simulink model "CalebsLaunchControl"  (R2019b)
settings: Solver=ode1  StartTime=0.0  StopTime=inf  FixedStep=0.0002  RelTol=1e-3
PreLoadFcn:
  | vehicle = 'Car'; if ~length(which('cmself')), cmenv; end
  | CalebsLaunchControl_bus
InitFcn:
  | vehicle = 'Car'; if ~length(which('cmself')), cmenv; end
  | CalebsLaunchControl_bus
model workspace (MAT data in the model file):
  LC_REVRANGE = [0 400 800 1200 1600 2000 3000 4000 6000 22000]
  MotorData = [0 4 8 13 17 21 0 4 8 13 17 21 ... (84 elements, 6x14)]
  POWER_AT_FULL_GAS = [21 21 21 21 21 21 21 21 21 20 20 19 ... (14 elements, 1x14)]
  RPM_RANGE = [0 2000 4000 6000 8000 10000 12000 14000 15000 16000 17000 18000 ... (14 elements, 1x14)]
  TC_MODE_ONE = [18 20 23 25 25 25 25 25 25 25]
  TC_MODE_ONE_FRONT = [9 10 12 15 25 25 25 25 25 25 25 25 ... (14 elements, 1x14)]
  ThrottleOpening = [0 0.2 0.4 0.6 0.8 1]
libraries: CarMaker4SL x8
(part 2 of 2)

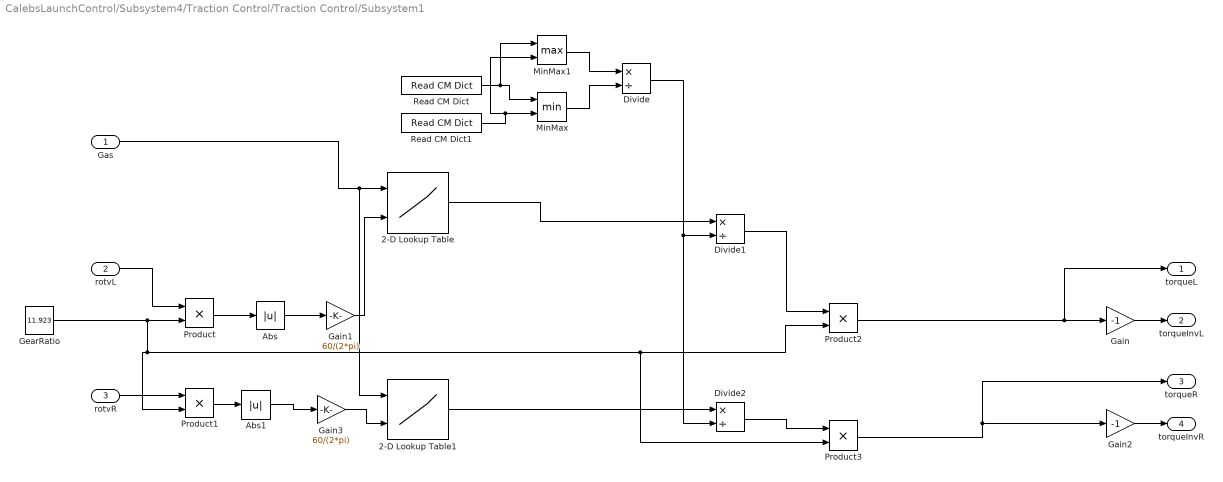
== system CalebsLaunchControl/Subsystem4/Traction Control/Traction Control/Subsystem1 ==
  Gas : Inport
  rotvL : Inport  Port=2
  rotvR : Inport  Port=3
  2-D Lookup Table : Lookup_n-D  BreakpointsForDimension1=ThrottleOpening  BreakpointsForDimension2=RPM_RANGE  Table=MotorData  InternalRulePriority=Speed  RndMeth=Simplest  InputSameDT=on
  2-D Lookup Table1 : Lookup_n-D  BreakpointsForDimension1=ThrottleOpening  BreakpointsForDimension2=RPM_RANGE  Table=MotorData  InternalRulePriority=Speed  RndMeth=Simplest  InputSameDT=on
  Abs : Abs
  Abs1 : Abs
  Divide : Product  Inputs=*/
  Divide1 : Product  Inputs=*/
  Divide2 : Product  Inputs=*/
  Gain : Gain  Gain=-1
  Gain1 : Gain  Gain=60/(2*pi)
  Gain2 : Gain  Gain=-1
  Gain3 : Gain  Gain=60/(2*pi)
  GearRatio : Constant  Value=11.923
  MinMax : MinMax  Inputs=2
  MinMax1 : MinMax  Function=max  Inputs=2
  Product{,1..3} (4 alike) : Product
  Read CM Dict : CarMaker4SL/Read CM Dict  xname=Car.LongSlipRL  xsync=off
  Read CM Dict1 : CarMaker4SL/Read CM Dict  xname=Car.LongSlipRR  xsync=off
  torqueL : Outport
  torqueInvL : Outport  Port=2
  torqueR : Outport  Port=3
  torqueInvR : Outport  Port=4
  wires:
  Gain/1 -> torqueInvL/1
  Product/1 -> Abs/1
  Gas/1 -> 2-D Lookup Table1/1, 2-D Lookup Table/1
  GearRatio/1 -> Product1/2, Product3/2, Product2/2, Product/2
  rotvL/1 -> Product/1
  Product2/1 -> Gain/1, torqueL/1
  Abs/1 -> Gain1/1
  Gain1/1 -> 2-D Lookup Table/2
  2-D Lookup Table/1 -> Divide1/1
  Gain2/1 -> torqueInvR/1
  Read CM Dict1/1 -> MinMax/2, MinMax1/2
  Read CM Dict/1 -> MinMax1/1, MinMax/1
  MinMax1/1 -> Divide/1
  MinMax/1 -> Divide/2
  Divide/1 -> Divide2/2, Divide1/2
  Divide1/1 -> Product2/1
  rotvR/1 -> Product1/1
  Gain3/1 -> 2-D Lookup Table1/2
  Product1/1 -> Abs1/1
  Abs1/1 -> Gain3/1
  2-D Lookup Table1/1 -> Divide2/1
  Divide2/1 -> Product3/1
  Product3/1 -> torqueR/1, Gain2/1

== system CalebsLaunchControl/Subsystem4/Launch Control/LaunchControl/Subsystem/If Action Subsystem ==
  In1 : Inport
  Action Port : ActionPort  ActionPortLabel=if(u2< u1)
  Out1 : Outport
  wires:
  In1/1 -> Out1/1

== system CalebsLaunchControl/Subsystem4/Launch Control/LaunchControl/Subsystem/If Action Subsystem1 ==
  In1 : Inport
  Action Port : ActionPort  ActionPortLabel=else
  Out1 : Outport
  wires:
  In1/1 -> Out1/1

== system CalebsLaunchControl/Subsystem4/Launch Control/LaunchControl/Subsystem1/If Action Subsystem ==
  In1 : Inport
  Action Port : ActionPort  ActionPortLabel=if(u2< u1)
  Out1 : Outport
  wires:
  In1/1 -> Out1/1

== system CalebsLaunchControl/Subsystem4/Launch Control/LaunchControl/Subsystem1/If Action Subsystem1 ==
  In1 : Inport
  Action Port : ActionPort  ActionPortLabel=else
  Out1 : Outport
  wires:
  In1/1 -> Out1/1

== system CalebsLaunchControl/Subsystem4/Launch Control/LaunchControl/Subsystem2/If Action Subsystem ==
  In1 : Inport
  Action Port : ActionPort  ActionPortLabel=if(u2< u1)
  Out1 : Outport
  wires:
  In1/1 -> Out1/1

== system CalebsLaunchControl/Subsystem4/Launch Control/LaunchControl/Subsystem2/If Action Subsystem1 ==
  In1 : Inport
  Action Port : ActionPort  ActionPortLabel=else
  Out1 : Outport
  wires:
  In1/1 -> Out1/1

== system CalebsLaunchControl/Subsystem4/Launch Control/LaunchControl/Subsystem3/If Action Subsystem ==
  In1 : Inport
  Action Port : ActionPort  ActionPortLabel=if(u2< u1)
  Out1 : Outport
  wires:
  In1/1 -> Out1/1

== system CalebsLaunchControl/Subsystem4/Launch Control/LaunchControl/Subsystem3/If Action Subsystem1 ==
  In1 : Inport
  Action Port : ActionPort  ActionPortLabel=else
  Out1 : Outport
  wires:
  In1/1 -> Out1/1
